simulink model "Beta_Estimation_KalmanFilter"  (R2022b)
settings: Solver=FixedStepAuto  StartTime=0.0  StopTime=t_l  FixedStep=0.001  RelTol=1e-3
values from neighbouring files (symbols this model uses):
  A = [-(2*Cf_nom+2*Cr_nom)/(M*Vel) (-1+(-2*Lf*Cf_nom+2*Lr*Cr_nom)/(M*Vel^2)) ;      (-2*Lf*Cf_nom + 2*Lr*Cr_nom)/J (-2*Lf^2*Cf_nom-2*Lr^2*Cr_nom)/(J*Vel)]    [State_Estimator.m]
  B = [2*Cf_nom/M/Vel ; 2*Lf*Cf_nom/J]    [State_Estimator.m]
  C = [0 1]    [State_Estimator.m]
  Time = data.X.Data'    [Cornering_Stiffness_Tuning.m]    (also in Lat_Dynamics_Simul_initialize.m = (0 : 0.001 : t_l)'; State_Estimator.m)
undefined symbols (not defined in the file or in its folder): Continuous
libraries: ctrlSharedLib x1
settings Model: Creator=LDW  LastModifiedBy=lego0

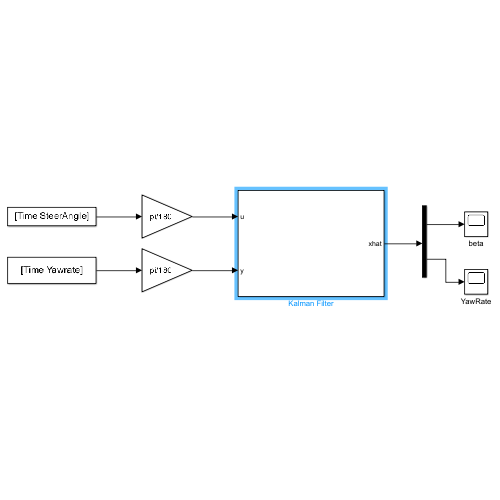
[thumbnail: Simulink's stored preview of the top-level diagram]
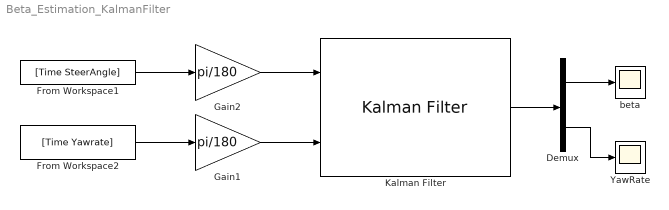
== system Beta_Estimation_KalmanFilter ==
  Demux : Demux  Outputs=2
  From Workspace1 : FromWorkspace  VariableName=[Time SteerAngle]
  From Workspace2 : FromWorkspace  VariableName=[Time Yawrate]
  Gain1 : Gain  Gain=pi/180
  Gain2 : Gain  Gain=pi/180
  Kalman Filter : ctrlSharedLib/Kalman Filter  TimeDomain=Continuous-Time  UseCurrentEstimator=on  ModelSource=Individual A, B, C, D matrices  ModelSourceVariable=ss(0.95,1,1,0,1)  A=A  B=B  C=C  D=0  NumberOfStates=1  NumberOfInputs=1  NumberOfOutputs=1  InitialEstimateSource=Dialog  X0=[0 ; 0]  P0=10  UseK=off  UseGH=off  NumberOfProcessNoiseInputs=1  G=1  TimeInvariantG=on  H=0  TimeInvariantH=on  Q=1  TimeInvariantQ=on  R=100  TimeInvariantR=on  N=0  TimeInvariantN=on  AddInputPort=on  AddEnablePort=off  OutputEstimatedY=off  OutputP=off  Ts=-1
  YawRate : Scope
  beta : Scope
  wires:
  From Workspace2/1 -> Gain1/1
  From Workspace1/1 -> Gain2/1
  Kalman Filter/1 -> Demux/1
  Demux/1 -> beta/1
  Demux/2 -> YawRate/1
  Gain2/1 -> Kalman Filter/1
  Gain1/1 -> Kalman Filter/2
